simulink model "ls_system"  (Simulink 3.00)
settings: Solver=ode45  StartTime=0.0  StopTime=100  FixedStep=0.01  MaxStep=0.01  RelTol=1e-3
undefined symbols (not defined in the file or in its folder): seed
settings Model: LastModifiedBy=administrator

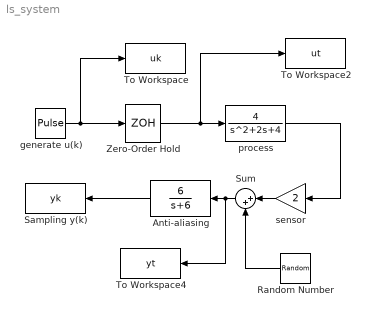
== system ls_system ==
  Anti-aliasing : TransferFcn  Orientation=left  Numerator=[6]  Denominator=[1 6]
  Random Number : RandomNumber  Orientation=left  Mean=0  Variance=0.00001  Seed=seed  SampleTime=0.01
  Sampling y(k) : ToWorkspace  VariableName=yk  SampleTime=0.5  SaveFormat=Matrix
  Sum : Sum  Orientation=left  Inputs=|++  SaturateOnIntegerOverflow=on
  To Workspace : ToWorkspace  VariableName=uk  SampleTime=0.5  SaveFormat=Matrix
  To Workspace2 : ToWorkspace  VariableName=ut  SampleTime=0.01  SaveFormat=Matrix
  To Workspace4 : ToWorkspace  VariableName=yt  SampleTime=0.01  SaveFormat=Matrix
  Zero-Order Hold : ZeroOrderHold  SampleTime=0.5
  generate u(k) : DiscretePulseGenerator  Amplitude=1  Period=30  PulseWidth=15  PhaseDelay=0  SampleTime=0.5
  process : TransferFcn  Numerator=[4]  Denominator=[1 2 4]
  sensor : Gain  Orientation=left  Gain=2  SaturateOnIntegerOverflow=on
  wires:
  generate u(k)/1 -> Zero-Order Hold/1, To Workspace/1
  Anti-aliasing/1 -> Sampling y(k)/1
  Zero-Order Hold/1 -> process/1, To Workspace2/1
  sensor/1 -> Sum/1
  Random Number/1 -> Sum/2
  Sum/1 -> Anti-aliasing/1, To Workspace4/1
  process/1 -> sensor/1
